simulink model "pfb_fir"  (Simulink 7.0)
settings: Solver=FixedStepDiscrete  SolverMode=SingleTasking  StartTime=0.0  StopTime=10.0  RelTol=1e-3
undefined symbols (not defined in the file): pfb_coefs
libraries: xbsIndex_r4 x385
(part 8 of 27)

== system pfb_fir/fir_2/fir_tap_1 ==
  data_in : Inport  OutDataType=sfix(16)  OutScaling=2^0
  sum_in : Inport  Port=2  OutDataType=sfix(16)  OutScaling=2^0
  sync_in : Inport  Port=3  OutDataType=sfix(16)  OutScaling=2^0
  fir_coef : Subsystem  mask(FIR Filter Coefficient Generator){coef=[7.55822333239443e-005;0.000226337373781674;0.000376546527419557;0.000526209439676531;0.000675325864794748;0.000823895565799559;0.000971918314479012;0.00111939389136366;0.00126632208570627;0.00141270269546109;0.00155853552726339;0.00170382039640892;0.00184855712683285;0.00199274555108931;0.00213638551033019;0.0022794768542842;0.00242201944123601;0.00256401313800475;0.00270545781992298;0.00284635337081542;0.00298669968297734;0.00312649665715319;0.00326574420251518;0.00340444223664131;0.00354259068549404;0.00368018948339813;0.00381723857301899;0.00395373790534074;0.00408968743964404;0.00422508714348402;0.00435993699266828;0.00449423697123439;0.00462798707142765;0.00476118729367882;0.00489383764658139;0.00502593814686929;0.00515748881939405;0.00528848969710218;0.00541894082101253;0.00554884224019323;0.00567819401173886;0.00580699620074764;0.00593524888029807;0.006062952131426;0.0061901060431015;0.00631671071220536;0.00644276624350604;0.00656827274963604;0.00669323035106852;0.00681763917609391;0.00694149936079604;0.00706481104902866;0.00718757439239176;0.00730978955020755;0.00743145668949677;0.00755257598495482;0.00767314761892755;0.00779317178138749;0.00791264866990946;0.00803157848964654;0.00814996145330591;0.00826779778112436;0.00838508770084402;0.00850183144768805;0.00861802926433593;0.00873368140089908;0.00884878811489629;0.00896334967122888;0.00907736634215623;0.00919083840727075;0.00930376615347321;0.0094161498749479;0.00952798987313748;0.00963928645671813;0.00975003994157455;0.00986025065077467;0.00996991891454458;0.0100790450702434;0.0101876294623378;0.0102956724423769;0.0104031743689668;0.010510135607745;0.0106165565313551;0.0107224375194214;0.0108277789585228;0.010932581242168;0.0110368447707688;0.0111405699516152;0.0112437571988492;0.0113464069334393;0.0114485195831541;0.0115500955825369;0.0116511353728793;0.0117516394021958;0.0118516081251968;0.0119510420032635;0.012049941504421;0.0121483071033125;0.0122461392811728;0.0123434385258024;0.0124402053315406;0.0125364401992397;0.0126321436362382;0.0127273161563346;0.0128219582797607;0.0129160705331552;0.0130096534495371;0.013102707568279;0.0131952334350806;0.0132872316019417;0.013378702627136;0.0134696470751837;0.0135600655168253;0.0136499585289943;0.0137393266947904;0.0138281706034528;0.0139164908503332;0.0140042880368685;0.0140915627705541;0.0141783156649169;0.0142645473394878;0.0143502584197752;0.014435449537237;0.0145201213292544;0.0146042744391039;0.0146879095159304;0.0147710272147199;0.014853628196272;0.014935713127173;0.0150172826797681;0.0150983375321339;0.0151788783680517;0.0152589058769791;0.0153384207540233;0.0154174236999132;0.0154959154209719;0.0155738966290892;0.015651368041694;0.0157283303817268;0.0158047843776117;0.0158807307632293;0.0159561702778886;0.0160311036662993;0.0161055316785444;0.016179455070052;0.0162528746015679;0.0163257910391276;0.0163982051540287;0.0164701177228029;0.0165415295271879;0.0166124413541001;0.0166828539956064;0.016752768248896;0.0168221849162531;0.0168911048050285;0.0169595287276116;0.0170274575014029;0.0170948919487855;0.0171618328970972;0.0172282811786028;0.0172942376304655;0.0173597030947194;0.0174246784182411;0.0174891644527217;0.0175531620546388;0.0176166720852282;0.0176796954104559;0.01774223290099;0.0178042854321725;0.0178658538839913;0.0179269391410516;0.0179875420925484;0.0180476636322377;0.0181073046584087;0.0181664660738554;0.0182251487858485;0.0182833537061072;0.018341081750771;0.0183983338403711;0.018455110899803;0.0185114138582973;0.0185672436493922;0.0186226012109047;0.0186774874849029;0.0187319034176773;0.0187858499597128;0.0188393280656603;0.0188923386943085;0.0189448828085557;0.0189969613753813;0.0190485753658179;0.0190997257549227;0.0191504135217495;0.0192006396493202;0.0192504051245967;0.0192997109384527;0.019348558085645;0.0193969475647859;0.0194448803783146;0.0194923575324687;0.0195393800372564;0.0195859489064282;0.0196320651574482;0.0196777298114666;0.0197229438932907;0.0197677084313573;0.0198120244577041 ...(+15786 chars)], n_bits_c=9, bin_pt_c=8, use_bram=on}
      mask prompts: coef "Tap Coefficient(s)"; n_bits_c "Number of Coefficient Bits"; bin_pt_c "Coefficient Binary Point"; use_bram "Use BRAM for Coefficients"
      mask help: A Finite Impluse Response filter coefficient generator. This FIR filter coefficient generator outputs real coefficients. It can output one coefficient or cycle through a vector of coefficients for WOLA (Weighted OverLap Add) FIR filters.
      settings: AttributesFormatString=1024 coefs in bram
      mask Help:
      | <pre>
      | Description::
      | 
      | A Finite Impluse Response filter coefficient generator.
      | This FIR filter coefficient generator outputs real coefficients.
      | It can output one coefficient or cycle through a vector of coefficients for WOLA
      | (Weighted OverLap Add) FIR filters.
      | 
      | Mask Parameters::
      | 
      | Tap Coefficiant(s) (coef): The coefficient(s) to output.  For a "regular" FIR filter, this will be a
      | single number.  For a WOLA (Weighted OverLap Add) filter, this will be a vector of numbers.
      | These should be specified as doubles.   They will be rounded and saturated according to the
      | specified number of bits (n_bits_c) and binary point (bin_pt_c).
      | 
      | Number of Coefficient Bits (n_bits_c): The number of bits used for the fixed point binary
      | representation of the coefficient(s).
      | 
      | Coefficient Binary Point (bin_pt_c): The binary point of the fixed point binary representation
      | of the coefficient(s).
      | 
      | Use BRAM for Coefficients (use_bram): Check this checkbox to store the coefficients in BRAM.
      | If unchecked, the coefficients will be stored in distributed memory (i.e. slices).
      | This is only relevant is length(coef) is greater than 1; otherwise, a constant block is used.
      | </pre>
  fir_core : Subsystem  mask(FIR Filter Core){delay=1024, n_bits_d=8, bin_pt_d=7, n_bits_s=17, bin_pt_s=15, use_bram=on, mult_latency=3, add_latency=1, add_bypass=on}
      mask prompts: delay "Tap Delay"; n_bits_d "Number of Data Bits"; bin_pt_d "Data Binary Point"; n_bits_s "Number of Sum Bits"; bin_pt_s "Sum Binary Point"; use_bram "Use BRAM for Delay"; mult_latency "Multiplier Latency"; add_latency "Adder Latency"; add_bypass "Bypass Adder"
      mask help: A Finite Impluse Response Filter core with complex inputs and real coefficients. This FIR filter core does not have provisions for folding the input sequence to improve multiplier efficiency, so it is suboptimal for "regular" (i.e. non-WOLA) FIR filters. It is intended primarily for WOLA (Weighted OverLap Add) FIR filters.
      settings: AttributesFormatString=delay 1024 in bram\nno adder
      mask Help:
      | <pre>
      | Description::
      | 
      | A Finite Impluse Response Filter core with complex inputs and real coefficients.
      | 
      | This Finite Impluse Response Filter core is designed to be paired with a FIR Coefficient Generator
      | to form a FIR filter tap.  This FIR filter core does not have provisions for folding the input
      | sequence to improve multiplier efficiency, so it is suboptimal for "regular" (i.e. non-WOLA)
      | FIR filters.  It is intended primarily for WOLA (Weighted OverLap Add) FIR filters.
      | 
      | Mask Parameters::
      | 
      | Tap Delay (delay):  The inter-tap delay (the N in "z^-N").  For a regular FIR filter, this will be 1.
      | 
      | Number of Data Bits (n_bits_d): The number of bits for real/imaginary components of the data.
      | 
      | Data Binary Point (bin_pt_d): The binary point for real/imaginary components of the data.
      | 
      | Number of Sum Bits (n_bits_s): Specifies the width of the sum (overflow wraps).
      | 
      | Sum Binary Point (bin_pt_s): Specifies the binary point of the sum (quantization truncates).
      | 
      | Use BRAM for Delay (use_bram): Check this checkbox to implement the delay using BRAM.
      | If unchecked, the delay will be implemented using SLR16 elements (i.e. slices).
      | 
      | Multiplier Latency (mult_latency): Latency to use for the underlying multiplier.
      | 
      | Adder Latency (add_latency): Latency to use for the underlying adder.
      | 
      | Adder Bypass (add_bypass): Check this checkbox to bypass the adder.
      | Typically used for the first tap of a multi-tap FIR filter.
      | </pre>
  data_out : Outport  OutDataType=sfix(16)  OutScaling=2^0
  sum_out : Outport  Port=2  OutDataType=sfix(16)  OutScaling=2^0
  sync_out : Outport  Port=3  OutDataType=sfix(16)  OutScaling=2^0
  wires:
  fir_core/3(sync_out) -> sync_out/1
  fir_core/2(sum_out) -> sum_out/1
  fir_core/1(data_out) -> data_out/1
  sync_in/1 -> fir_coef/3(sync_in)
  sum_in/1 -> fir_coef/2(sum_in)
  data_in/1 -> fir_coef/1(data_in)
  fir_coef/4(sync_out) -> fir_core/4(sync_in)
  fir_coef/3(coef) -> fir_core/3(coef)
  fir_coef/2(sum_out) -> fir_core/2(sum_in)
  fir_coef/1(data_out) -> fir_core/1(data_in)
